simulink model "relop_complex_test"  (Simulink 8.4)
settings: Solver=ode45  StartTime=0.0  StopTime=10.0  RelTol=1e-3
settings Model: Creator=arnaud  LastModifiedBy=arnaud

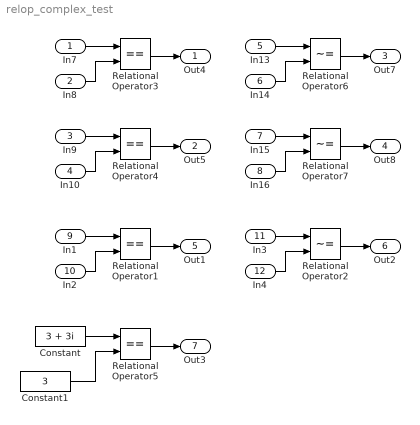
== system relop_complex_test ==
  In7 : Inport  OutDataTypeStr=double  PortDimensions=1
      settings: SignalType=complex
  In8 : Inport  Port=2  OutDataTypeStr=double  PortDimensions=1
      settings: SignalType=complex
  In9 : Inport  Port=3  OutDataTypeStr=int8  PortDimensions=1
      settings: SignalType=complex
  In10 : Inport  Port=4  OutDataTypeStr=int8  PortDimensions=1
      settings: SignalType=complex
  In13 : Inport  Port=5  OutDataTypeStr=double
      settings: SignalType=complex
  In14 : Inport  Port=6  OutDataTypeStr=double
      settings: SignalType=complex
  In15 : Inport  Port=7  OutDataTypeStr=int8
      settings: SignalType=complex
  In16 : Inport  Port=8  OutDataTypeStr=int8
      settings: SignalType=complex
  In1 : Inport  Port=9  OutDataTypeStr=double  PortDimensions=1
      settings: SignalType=complex
  In2 : Inport  Port=10  OutDataTypeStr=double  PortDimensions=1
  In3 : Inport  Port=11  OutDataTypeStr=double
  In4 : Inport  Port=12  OutDataTypeStr=double
      settings: SignalType=complex
  Constant : Constant  Value=3 + 3i
  Constant1 : Constant  Value=3
  Relational Operator{1,3..5} (4 alike) : RelationalOperator  Operator===  OutDataTypeStr=boolean
  Relational Operator2 : RelationalOperator  Operator=~=  OutDataTypeStr=boolean
  Relational Operator6 : RelationalOperator  Operator=~=  OutDataTypeStr=boolean
  Relational Operator7 : RelationalOperator  Operator=~=  OutDataTypeStr=boolean
  Out4 : Outport
  Out5 : Outport  Port=2
  Out7 : Outport  Port=3
  Out8 : Outport  Port=4
  Out1 : Outport  Port=5
  Out2 : Outport  Port=6
  Out3 : Outport  Port=7
  wires:
  In7/1 -> Relational Operator3/1
  Relational Operator3/1 -> Out4/1
  In8/1 -> Relational Operator3/2
  In9/1 -> Relational Operator4/1
  Relational Operator4/1 -> Out5/1
  In10/1 -> Relational Operator4/2
  In13/1 -> Relational Operator6/1
  Relational Operator6/1 -> Out7/1
  In14/1 -> Relational Operator6/2
  In15/1 -> Relational Operator7/1
  Relational Operator7/1 -> Out8/1
  In16/1 -> Relational Operator7/2
  In1/1 -> Relational Operator1/1
  Relational Operator1/1 -> Out1/1
  In2/1 -> Relational Operator1/2
  In3/1 -> Relational Operator2/1
  Relational Operator2/1 -> Out2/1
  In4/1 -> Relational Operator2/2
  Constant/1 -> Relational Operator5/1
  Relational Operator5/1 -> Out3/1
  Constant1/1 -> Relational Operator5/2
